simulink model "Exercitiul2"  (R2016a)
settings: Solver=VariableStepAuto  StartTime=0.0  StopTime=10  RelTol=1e-3
undefined symbols (not defined in the file): m
settings Model: Creator=Cristina  LastModifiedBy=Cristina

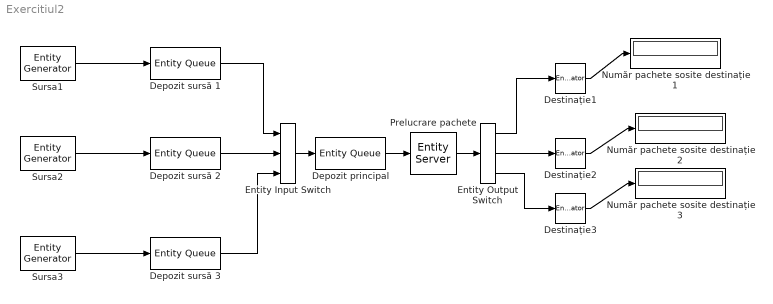
== system Exercitiul2 ==
  Depozit principal : EntityQueue  InputPortMessageModes=m  OutputPortMessageModes=m
      settings: OutputPortMap=o5
  Depozit sursă 1 : EntityQueue  InputPortMessageModes=m  OutputPortMessageModes=m
      settings: OutputPortMap=o5
  Depozit sursă 2 : EntityQueue  InputPortMessageModes=m  OutputPortMessageModes=m
      settings: OutputPortMap=o5
  Depozit sursă 3 : EntityQueue  InputPortMessageModes=m  OutputPortMessageModes=m
      settings: OutputPortMap=o5
  Destinație1 : EntityTerminator  InputPortMessageModes=m  NumberEntitiesArrived=on
      settings: OutputPortMap=o0
  Destinație2 : EntityTerminator  InputPortMessageModes=m  NumberEntitiesArrived=on
      settings: OutputPortMap=o0
  Destinație3 : EntityTerminator  InputPortMessageModes=m  NumberEntitiesArrived=on
      settings: OutputPortMap=o0
  Entity Input Switch : EntityInputSwitch  InputPortMessageModes=m,m,m  OutputPortMessageModes=m  NumberInputPorts=3
      settings: InputPortMap=u1,u2,u3
  Entity Output Switch : EntityOutputSwitch  InputPortMessageModes=m  OutputPortMessageModes=m,m,m  NumberOutputPorts=3  SwitchingCriterion=From attribute  SwitchAttributeName=IPdestinatie
      settings: OutputPortMap=o0,o1,o2
  Număr pachete sosite destinație 1 : Display
  Număr pachete sosite destinație 2 : Display
  Număr pachete sosite destinație 3 : Display
  "Prelucrare pachete " : EntityServer  InputPortMessageModes=m  OutputPortMessageModes=m  Capacity=1  ServiceTimeSource=Attribute  ServiceTimeAttributeName=lungimeDate
  Sursa1 : EntityGenerator  OutputPortMessageModes=m  TimeSource=MATLAB action  IntergenerationTimeAction=|  AttributeName=IPsursa|IPdestinatie|lungimeDate  AttributeInitialValue=1|3|6 + 4 * rand  EntityType=Structured  EntityTypeName=Entity
      | persistent init
      | if (isempty(init))
      |     rng(122);
      |     init = true;
      | end
      | dt = exprnd(0.008);
  Sursa2 : EntityGenerator  OutputPortMessageModes=m  TimeSource=MATLAB action  IntergenerationTimeAction=|  AttributeName=IPsursa|IPdestinatie|lungimeDate  AttributeInitialValue=2|1|6 + 4 * rand  EntityType=Structured  EntityTypeName=Entity
      | persistent init
      | if (isempty(init))
      |     rng(123);
      |     init = true;
      | end
      | dt = exprnd(0.008);
  Sursa3 : EntityGenerator  OutputPortMessageModes=m  TimeSource=MATLAB action  IntergenerationTimeAction=|  AttributeName=IPsursa|IPdestinatie|lungimeDate  AttributeInitialValue=3|2|6 + 4 * rand  EntityType=Structured  EntityTypeName=Entity
      | persistent init
      | if (isempty(init))
      |     rng(125);
      |     init = true;
      | end
      | dt = exprnd(0.008);
  wires:
  Sursa1/1 -> Depozit sursă 1/1
  Depozit sursă 1/1 -> Entity Input Switch/1
  Depozit sursă 2/1 -> Entity Input Switch/2
  Depozit sursă 3/1 -> Entity Input Switch/3
  Sursa2/1 -> Depozit sursă 2/1
  Sursa3/1 -> Depozit sursă 3/1
  Entity Input Switch/1 -> Depozit principal/1
  Entity Output Switch/1 -> Destinație1/1
  Entity Output Switch/2 -> Destinație2/1
  Entity Output Switch/3 -> Destinație3/1
  "Prelucrare pachete "/1 -> Entity Output Switch/1
  Destinație1/1 -> Număr pachete sosite destinație 1/1
  Destinație2/1 -> Număr pachete sosite destinație 2/1
  Destinație3/1 -> Număr pachete sosite destinație 3/1
  Depozit principal/1 -> "Prelucrare pachete "/1
